simulink model "Trial"  (R2024b)
settings: Solver=VariableStepAuto  StartTime=0.0  StopTime=0.0002  RelTol=1e-3
PreLoadFcn:
  | System
values from neighbouring files (symbols this model uses):
  Fs = 300e6    (= 300000000)    [IFM.m]    (also in System.m; SystemInput.m = p.Results.Fs)
  JustNoiseSamples = Fs*JustNoiseTime    (= 30000)    [IFM.m]    (also in System.m; SystemInput.m = Fs * 100e-6)
libraries: hdlBasic x18, vmcUtilities x1
settings Model: Creator=fsy  LastModifiedBy=fsydere

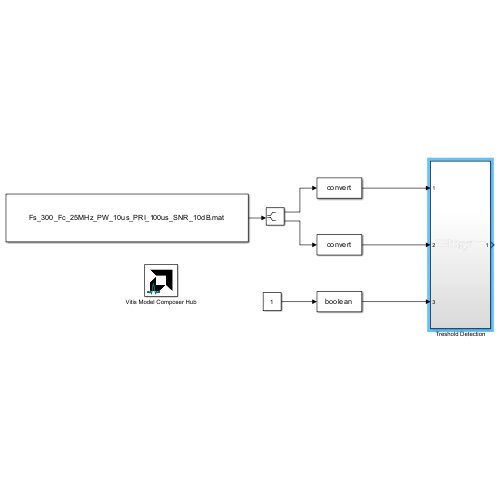
[thumbnail: Simulink's stored preview of the top-level diagram]
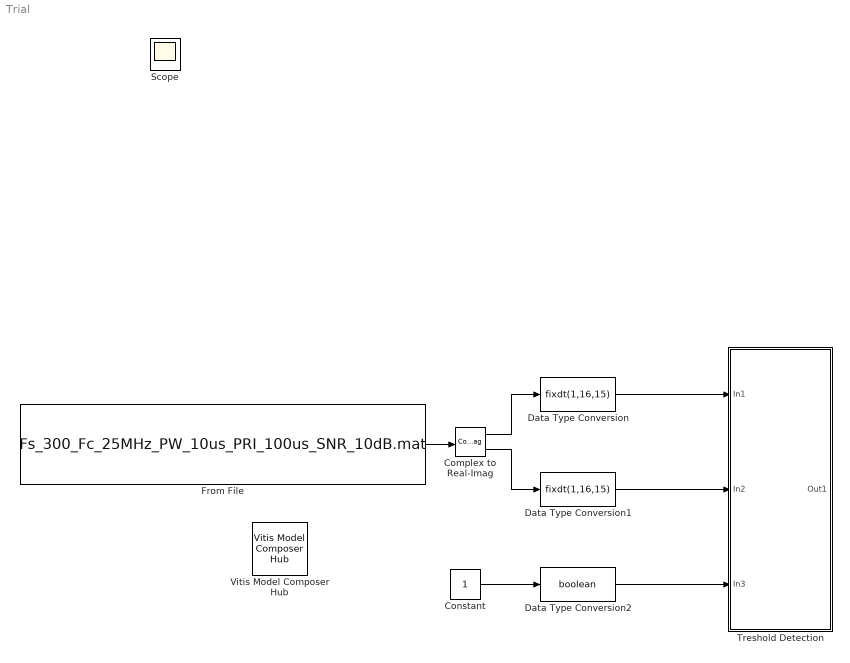
== system Trial ==
  Complex to Real-Imag : ComplexToRealImag
  Constant : Constant  SampleTime=1/Fs
  Data Type Conversion : DataTypeConversion  OutDataTypeStr=fixdt(1,16,15)  RndMeth=Round
  Data Type Conversion1 : DataTypeConversion  OutDataTypeStr=fixdt(1,16,15)  RndMeth=Round
  Data Type Conversion2 : DataTypeConversion  OutDataTypeStr=boolean  RndMeth=Round
  From File : FromFile  FileName=Fs_300_Fc_25MHz_PW_10us_PRI_100us_SNR_10dB.mat  SampleTime=1/Fs
  Treshold Detection : Subsystem
  Vitis Model Composer Hub : vmcUtilities/Vitis Model Composer Hub  Tag=genX  CodeGeneration=off  SubsystemName=Treshold Detection  CompilationType=HDLCompilation  ExportTypeV2=IP Catalog  StartColumn=1  NumberOfColumns=1  TargetDirectory=./netlist  exportDesign=off  analyzeDesign=off  validateDesignOnHw=off  ExportType=AI Engines  IpVendor=xilinx.com  IpLibrary=hls  IpVersion=1.0  IpHWLanguage=Verilog  AieCompilerOptions={}  AieSimulatorOptions={}  CreateTestbench=off  TestbenchStackSize=10  RunRtlSim=off  RunCSim=off  RunAieSim=off  AieSimTimeout=50000  RunAieSimProfiling=off  LaunchVitisAnalyzer=off  PlotOutput=off  RunX86Sim=off  X86SimTimeout=10  GenHwImage=off  GenLibadfXo=on  GenHwValidationCode=off  PlatformType=Not Specified  HwSystemType=Baremetal  HwValidationTarget=hw  ProjDevice=Zynq UltraScale+ ZCU102 Evaluation Board (xczu9eg-ffvb1156-2-e)  ProjDevicePart=xczu9eg-ffvb1156-2-e  AIEType=None  SamplePeriod=-1  ClockFrequency=200  DataPathParallelism=1  xilinxfamily=zynquplus  part=xczu9eg  speed=-2-e  package=ffvb1156  directory=./netlist/ip/Treshold_Detection/src  testbench=off  incr_netlist=off  synthesis_tool=Vivado  clock_wrapper=Clock Enables  dbl_ovrd=According to Block Masks  dcm_input_clock_period=10  sysclk_period=1e9/Fs  simulink_period=1/Fs  eval_field=0  LogFileName=''  NThreads=4
  Scope : Scope
  wires:
  From File/1 -> Complex to Real-Imag/1
  Complex to Real-Imag/2 -> Data Type Conversion1/1
  Complex to Real-Imag/1 -> Data Type Conversion/1
  Constant/1 -> Data Type Conversion2/1
  Data Type Conversion/1 -> Treshold Detection/1(In1)
  Data Type Conversion1/1 -> Treshold Detection/2(In2)
  Data Type Conversion2/1 -> Treshold Detection/3(In3)

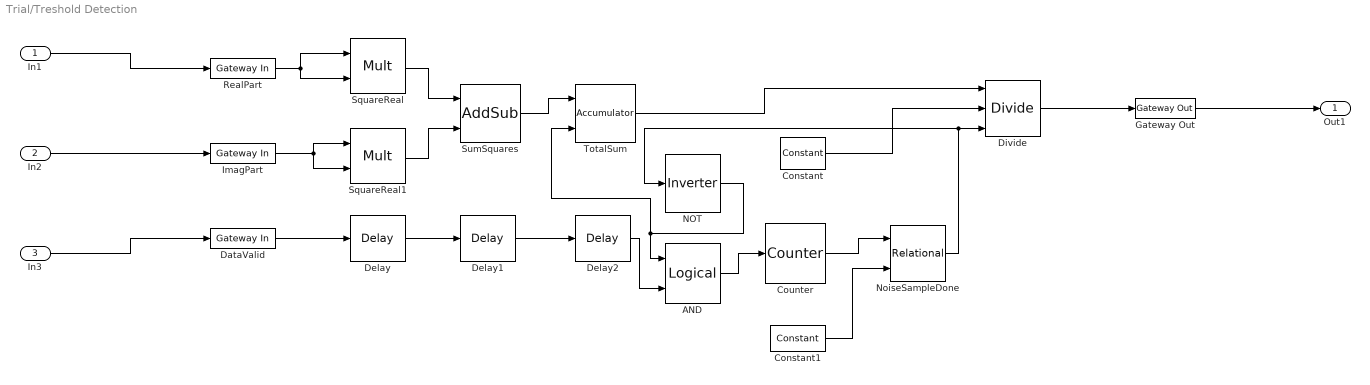
== system Trial/Treshold Detection ==
  In1 : Inport
  In2 : Inport  Port=2
  In3 : Inport  Port=3
  AND : hdlBasic/Logical  logical_function=AND  inputs=2  en=off  latency=0  precision=Full  arith_type=Unsigned  n_bits=16  bin_pt=0  align_bp=on  overflow=[]  quantization=[]  XmcBlockStatus=1  maskContainerNames=tabcontainer1  block_type=logical  block_config=sysgen:Logical_config
  Constant : hdlBasic/Constant  const=JustNoiseSamples  gui_display_data_type=Fixed-point  arith_type=Unsigned  n_bits=48  bin_pt=30  preci_type=Single  exp_width=8  frac_width=24  explicit_period=off  period=1  XmcBlockStatus=1  maskContainerNames=tabcontainer1  block_type=constant  block_config=sysgen:Constant_config
  Constant1 : hdlBasic/Constant  const=JustNoiseSamples-1  gui_display_data_type=Fixed-point  arith_type=Unsigned  n_bits=15  bin_pt=0  preci_type=Single  exp_width=8  frac_width=24  explicit_period=off  period=1  XmcBlockStatus=1  maskContainerNames=tabcontainer1  block_type=constant  block_config=sysgen:Constant_config
  Counter : hdlBasic/Counter  cnt_type=Count limited  cnt_to=JustNoiseSamples-1  operation=Up  start_count=0  cnt_by_val=1  arith_type=Unsigned  n_bits=15  bin_pt=0  load_pin=off  rst=off  en=on  explicit_period=Explicit  period=1/Fs  use_behavioral_HDL=off  implementation=Fabric  XmcBlockStatus=1  maskContainerNames=group1  block_type=counter  block_config=sysgen:Counter_config  block_width=531  block_height=1023
  DataValid : hdlBasic/Gateway In  gui_display_data_type=Boolean  arith_type=Boolean  n_bits=16  bin_pt=15  preci_type=Single  exp_width=8  frac_width=24  rows=1  columns=1  quantization="Round  (unbiased: +/- Inf)"  overflow=Saturate  period=1/Fs  UseAsADC=off  ADCChannel='1'  interface=None  automatic_assignment=on  address_offset=hex2dec('00')  intf_name=''  intf_description=''  default_value=0  timing_constraint=None  locs_specified=off  LOCs={}  io_standard={}  inherit_from_input=off  hdl_port=on  XmcBlockStatus=1  maskContainerNames=group4  block_type=gatewayin  block_config=sysgen:gateway_in_config  block_width_w=590  block_height_w=620  block_width=640  block_height=850
  Delay : hdlBasic/Delay  rst=off  en=off  latency=3  reg_retiming=on  XmcBlockStatus=1  maskContainerNames=group1  block_type=delay  block_config=sysgen:Delay_config
  Delay1 : hdlBasic/Delay  rst=off  en=off  latency=1  reg_retiming=on  XmcBlockStatus=1  maskContainerNames=group1  block_type=delay  block_config=sysgen:Delay_config
  Delay2 : hdlBasic/Delay  rst=off  en=off  latency=1  reg_retiming=on  XmcBlockStatus=1  maskContainerNames=group1  block_type=delay  block_config=sysgen:Delay_config
  Divide : hdlBasic/Divide  flow_control=NonBlocking  axi_optimize_goal=Resources  algorithm_type=Radix2  fractional_width=30  latency=1  rate=1  has_a_tlast=off  has_a_tuser=off  has_b_tlast=off  has_b_tuser=off  en=on  has_result_tready=off  result_tlast_behv=Pass_A_TLAST  has_underflow=off  has_overflow=off  has_invalid_op=off  has_divide_by_zero=off  fpo_op_type=mergeddivide  XmcBlockStatus=1  maskContainerNames=tabcontainer1  block_type=divide  block_config=sysgen:FPOBlockDescriptor_config
  Gateway Out : hdlBasic/Gateway Out  inherit_from_input=on  bool_to_boolean=off  hdl_port=off  rows=1  columns=1  UseAsDAC=off  DACChannel='1'  interface=None  automatic_assignment=on  address_offset=hex2dec('00')  intf_name=''  intf_description=''  timing_constraint=None  locs_specified=off  LOCs={}  io_standard={}  XmcBlockStatus=1  maskContainerNames=group4  block_type=gatewayout  block_config=sysgen:gateway_out_config  block_width_w=590  block_height_w=620  block_width=620  block_height=750
  ImagPart : hdlBasic/Gateway In  gui_display_data_type=Fixed-point  arith_type=Signed (2's comp)  n_bits=16  bin_pt=15  preci_type=Single  exp_width=8  frac_width=24  rows=1  columns=1  quantization="Round  (unbiased: +/- Inf)"  overflow=Saturate  period=1/Fs  UseAsADC=off  ADCChannel='1'  interface=None  automatic_assignment=on  address_offset=hex2dec('00')  intf_name=''  intf_description=''  default_value=0  timing_constraint=None  locs_specified=off  LOCs={}  io_standard={}  inherit_from_input=off  hdl_port=on  XmcBlockStatus=1  maskContainerNames=group4  block_type=gatewayin  block_config=sysgen:gateway_in_config  block_width_w=590  block_height_w=620  block_width=640  block_height=850
  NOT : hdlBasic/Inverter  en=off  latency=0  XmcBlockStatus=1  maskContainerNames=group2  block_type=inv  block_config=sysgen:Inverter_config
  NoiseSampleDone : hdlBasic/Relational  mode=a=b  op_type=Bool  en=off  latency=0  XmcBlockStatus=1  maskContainerNames=tabcontainer1  block_type=relational  block_config=sysgen:Relational_config
  RealPart : hdlBasic/Gateway In  gui_display_data_type=Fixed-point  arith_type=Signed (2's comp)  n_bits=16  bin_pt=15  preci_type=Single  exp_width=8  frac_width=24  rows=1  columns=1  quantization="Round  (unbiased: +/- Inf)"  overflow=Saturate  period=1/Fs  UseAsADC=off  ADCChannel='1'  interface=None  automatic_assignment=on  address_offset=hex2dec('00')  intf_name=''  intf_description=''  default_value=0  timing_constraint=None  locs_specified=off  LOCs={}  io_standard={}  inherit_from_input=off  hdl_port=on  XmcBlockStatus=1  maskContainerNames=group4  block_type=gatewayin  block_config=sysgen:gateway_in_config  block_width_w=590  block_height_w=620  block_width=640  block_height=850
  SquareReal : hdlBasic/Mult  precision=User Defined  arith_type="Signed  (2's comp)"  n_bits=32  bin_pt=30  quantization="Round  (unbiased: +/- Inf)"  overflow=Saturate  en=off  latency=3  opt_float=off  fp_mult_usage=No Usage  use_behavioral_HDL=on  opt=Speed  use_embedded=on  optimum_pipeline=off  pipeline=on  use_rpm=on  placement_style=Triangular  XmcBlockStatus=1  maskContainerNames=group1  block_type=mult  block_config=sysgen:Mult_config  block_width=598  block_height=876
  SquareReal1 : hdlBasic/Mult  precision=User Defined  arith_type="Signed  (2's comp)"  n_bits=32  bin_pt=30  quantization="Round  (unbiased: +/- Inf)"  overflow=Saturate  en=off  latency=3  opt_float=off  fp_mult_usage=No Usage  use_behavioral_HDL=on  opt=Speed  use_embedded=on  optimum_pipeline=off  pipeline=on  use_rpm=on  placement_style=Triangular  XmcBlockStatus=1  maskContainerNames=group1  block_type=mult  block_config=sysgen:Mult_config  block_width=598  block_height=876
  SumSquares : hdlBasic/AddSub  mode=Addition  use_carryin=off  use_carryout=off  en=off  latency=1  precision=User Defined  arith_type=Unsigned  n_bits=32  bin_pt=30  quantization="Round  (unbiased: +/- Inf)"  overflow=Saturate  use_behavioral_HDL=off  hw_selection=Fabric  pipelined=off  XmcBlockStatus=1  maskContainerNames=tabcontainer1  block_type=addsub  block_config=sysgen:Addsub_config
  TotalSum : hdlBasic/Accumulator  operation=Add  n_bits=48  overflow=Flag as error  scale=1  rst=off  hasbypass=off  en=on  latency=1  msb_inp=33  msb=48  lsb=0  use_behavioral_HDL=on  implementation=Fabric  XmcBlockStatus=1  maskContainerNames=group3  block_type=accum  block_config=sysgen:Accum_config  block_width=566  block_height=845
  Out1 : Outport
  wires:
  SquareReal/1 -> SumSquares/1
  Constant1/1 -> NoiseSampleDone/2
  Counter/1 -> NoiseSampleDone/1
  In3/1 -> DataValid/1
  AND/1 -> Counter/1
  In1/1 -> RealPart/1
  NoiseSampleDone/1 -> Divide/3, NOT/1
  SumSquares/1 -> TotalSum/1
  Delay/1 -> Delay1/1
  Delay2/1 -> AND/2
  DataValid/1 -> Delay/1
  SquareReal1/1 -> SumSquares/2
  Delay1/1 -> Delay2/1
  NOT/1 -> TotalSum/2, AND/1
  Gateway Out/1 -> Out1/1
  RealPart/1 -> SquareReal/1, SquareReal/2
  ImagPart/1 -> SquareReal1/2, SquareReal1/1
  In2/1 -> ImagPart/1
  TotalSum/1 -> Divide/1
  Divide/1 -> Gateway Out/1
  Constant/1 -> Divide/2
